simulink model "SG__MDL_LOG_ISSUE"  (R2022b)
settings: Solver=FixedStepAuto  StartTime=0.0  StopTime=Inf  FixedStep=ts  RelTol=1e-3  EnableMultiTasking=on
model workspace (MAT data in the model file):
  N_trig = Simulink.Parameter
  N_trig.Value = 4
  N_trig.Description = 'number of samples for triggered pulse for recording'
  N_trig.DataType = 'auto'
  N_trig.Complexity = 'real'
  N_trig.Dimensions = [1 1]
  Sig = Simulink.Signal
  Sig.DataType = 'auto'
  Sig.Dimensions = -1
  Sig.DimensionsMode = 'auto'
  Sig.Complexity = 'auto'
  Sig.SampleTime = -1
  Sig.SamplingMode = 'auto'
  dtf_a = Simulink.Parameter
  dtf_a.Value = [1  1  1; 1  1  1; 1  1  1; 1  1  1; 1  1  1; 1  1  1; 1  1  1; 1  1  1; 1  1  1; 1  1  1; 1  1  1; 1  1  1; 1  1  1; 1  1  1; 1  1  1; 1  1  1]
  dtf_a.DataType = 'auto'
  dtf_a.Complexity = 'real'
  dtf_a.Dimensions = [16 3]
  dtf_b = Simulink.Parameter
  dtf_b.Value = [0.5  0.5  0.5; 0.5  0.5  0.5; 0.5  0.5  0.5; 0.5  0.5  0.5; 0.5  0.5  0.5; 0.5  0.5  0.5; 0.5  0.5  0.5; 0.5  0.5  0.5; 0.5  0.5  0.5; 0.5  0.5  0.5; 0.5  0.5  0.5; 0.5  0.5  0.5; 0.5  0.5  0.5; 0.5  0.5  0.5; 0.5  0.5  0.5; 0.5  0.5  0.5]
  dtf_b.DataType = 'auto'
  dtf_b.Complexity = 'real'
  dtf_b.Dimensions = [16 3]
  enable_source = Simulink.Parameter
  enable_source.Value = 0
  enable_source.DataType = 'boolean'
  enable_source.Complexity = 'real'
  enable_source.Dimensions = [1 1]
  freq_fin = Simulink.Parameter
  freq_fin.Value = 1200
  freq_fin.DataType = 'auto'
  freq_fin.Complexity = 'real'
  freq_fin.Dimensions = [1 1]
  freq_ini = Simulink.Parameter
  freq_ini.Value = 150
  freq_ini.DataType = 'auto'
  freq_ini.Complexity = 'real'
  freq_ini.Dimensions = [1 1]
  k_L = Simulink.Parameter
  k_L.Value = [0; 0; 0; 0; 0; 0; 0; 0; 0; 0; 0; 0; 0; 0; 0; 0]
  k_L.Description = 'Coupling on left of ER. [Linear, NL]'
  k_L.DataType = 'auto'
  k_L.Complexity = 'real'
  k_L.Dimensions = [16 1]
  k_L_NL = Simulink.Parameter
  k_L_NL.Value = [0; 0; 0; 0; 0; 0; 0; 0; 0; 0; 0; 0; 0; 0; 0; 0]
  k_L_NL.Description = 'Coupling on left of ER. [Linear, NL]'
  k_L_NL.DataType = 'auto'
  k_L_NL.Complexity = 'real'
  k_L_NL.Dimensions = [16 1]
  k_O_NL = Simulink.Parameter
  k_O_NL.Value = [0; 0; 0; 0; 0; 0; 0; 0; 0; 0; 0; 0; 0; 0; 0; 0]
  k_O_NL.Description = 'Onsite nonlinearity'
  k_O_NL.DataType = 'auto'
  k_O_NL.Complexity = 'real'
  k_O_NL.Dimensions = [16 1]
  k_R = Simulink.Parameter
  k_R.Value = [0; 0; 0; 0; 0; 0; 0; 0; 0; 0; 0; 0; 0; 0; 0; 0]
  k_R.Description = 'Coupling on right of ER. [Linear, NL]'
  k_R.DataType = 'auto'
  k_R.Complexity = 'real'
  k_R.Dimensions = [16 1]
  k_R_NL = Simulink.Parameter
  k_R_NL.Value = [0; 0; 0; 0; 0; 0; 0; 0; 0; 0; 0; 0; 0; 0; 0; 0]
  k_R_NL.Description = 'Coupling on right of ER. [Linear, NL]'
  k_R_NL.DataType = 'auto'
  k_R_NL.Complexity = 'real'
  k_R_NL.Dimensions = [16 1]
  rec = Simulink.Parameter
  rec.Value = 1
  rec.DataType = 'boolean'
  rec.Complexity = 'real'
  rec.Dimensions = [1 1]
  src_select = Simulink.Parameter
  src_select.Value = 0
  src_select.DataType = 'auto'
  src_select.Complexity = 'real'
  src_select.Dimensions = [1 1]
  sweep_gain = Simulink.Parameter
  sweep_gain.Value = 0.02
  sweep_gain.DataType = 'auto'
  sweep_gain.Complexity = 'real'
  sweep_gain.Dimensions = [1 1]
  tmax = Simulink.Parameter
  tmax.Value = 10
  tmax.DataType = 'auto'
  tmax.Complexity = 'real'
  tmax.Dimensions = [1 1]
  ts_rec = Simulink.Parameter
  ts_rec.Value = 0.0001
  ts_rec.DataType = 'auto'
  ts_rec.Complexity = 'real'
  ts_rec.Dimensions = [1 1]
values from neighbouring files (symbols this model uses):
  ts = 400e-6    (= 0.0004)    [StartScript.m]
libraries: slrealtimeloglib x3, simulink x2, hdlsllib x2
settings Model: SimulationMode=external  ExplicitPartitioning=on  DataflowThreadingImplementation=Pthreads  Creator=padlewsk  LastModifiedBy=padlewsk
settings SolverCC: AllowMultiTaskInputOutput=on  ConcurrentTasks=on  AlgebraicLoopSolver=TrustRegion  PositivePriorityOrder=on  AutoInsertRateTranBlk=on
settings DataIOCC: SaveFormat=StructureWithTime
settings OptimizationCC: GainParamInheritBuiltInType=on  RollThreshold=33  EfficientFloat2IntCast=on  SimCompilerOptimization=on
settings DebuggingCC: TasksWithSamePriorityMsg=none  UnconnectedInputMsg=warning  UnconnectedOutputMsg=warning  UnconnectedLineMsg=warning  ModelReferenceSymbolNameMessage=none
settings HardwareCC: ProdBitPerLong=64  ProdLongLongMode=on  ProdHWDeviceType=Intel->x86-64 (Linux 64)
settings ModelReferenceCC: EnableRefExpFcnMdlSchedulingChecks=on
settings RTWCC: Description=Simulink Real-Time  SystemTargetFile=slrealtime.tlc  TemplateMakefile=slrealtime_default_tmf  Toolchain=Simulink Real-Time Toolchain  BuildConfiguration=Faster Runs  CodeExecutionProfiling=on  TargetLang=C++
settings SimulinkRealTimeTargetCC: UseGCCFastMath=on

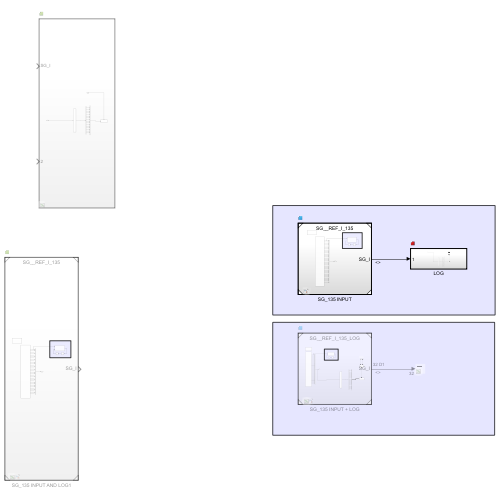
[thumbnail: Simulink's stored preview of the top-level diagram]
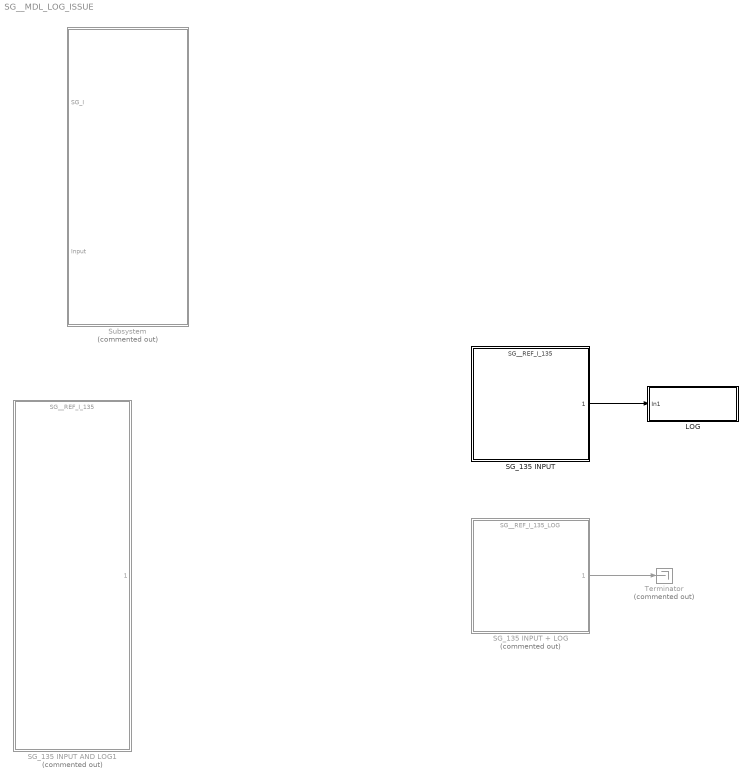
== system SG__MDL_LOG_ISSUE ==
  LOG : Subsystem  TreatAsAtomicUnit=on
  SG_135 INPUT : ModelReference  ModelNameDialog=SG__REF_I_135.slx  SimulationMode=Normal  ModelReferenceVersion=6.288
  SG_135 INPUT + LOG : ModelReference  Commented=on  ModelNameDialog=SG__REF_I_135_LOG.slx  SimulationMode=Normal  ModelReferenceVersion=6.291
  SG_135 INPUT AND LOG1 : ModelReference  Commented=on  ModelNameDialog=SG__REF_I_135.slx  SimulationMode=Normal  ModelReferenceVersion=6.288
  Subsystem : Subsystem  Commented=on  TreatAsAtomicUnit=on
  Terminator : Terminator  Commented=on
  wires:
  SG_135 INPUT/1 -> LOG/1(In1)
  SG_135 INPUT + LOG/1 -> Terminator/1

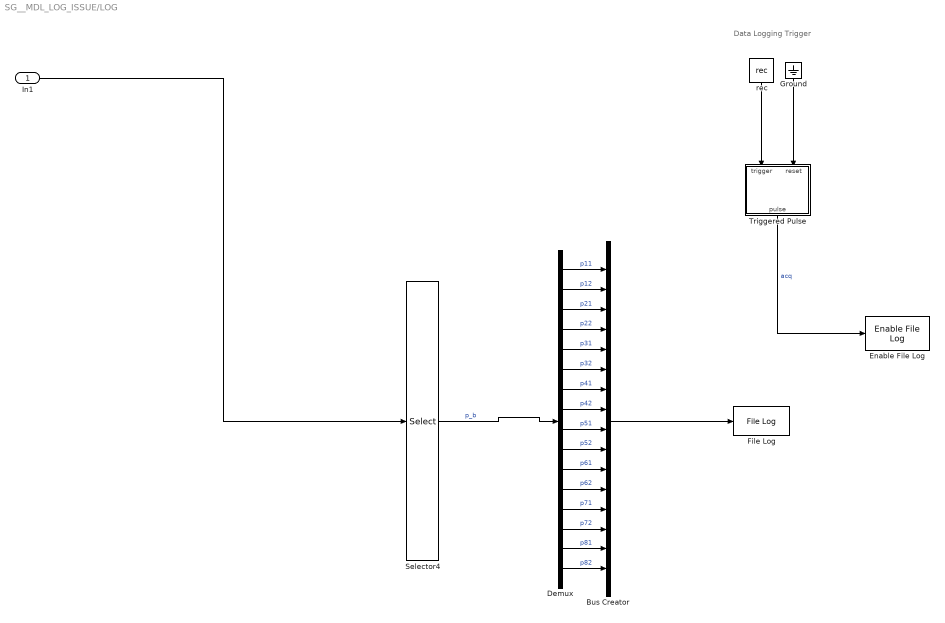
== system SG__MDL_LOG_ISSUE/LOG ==
  note: Data Logging Trigger
  In1 : Inport
  Bus Creator : BusCreator  Inputs=16
  Demux : Demux  Outputs=16
  Enable File Log : slrealtimeloglib/Enable File Log
  File Log : slrealtimeloglib/File Log  decimation=1  inputProcessing=Elements as channels (sample based)
  Ground : Ground
  Selector4 : Selector  InputPortWidth=32  IndexOptions=Index vector (dialog)  Indices=[1:2:32]  OutputSizes=1
  "Triggered Pulse " : Subsystem  TreatAsAtomicUnit=on  mask(Triggered Pulse){N=3000}
      mask prompts: N "Length (N samples)"
      mask help: Generates a single pulse of N samples length
  rec : Constant  Value=rec  SampleTime=-1
  wires:
  Demux/14 -> Bus Creator/14  "p72"
  Demux/10 -> Bus Creator/10  "p52"
  Demux/13 -> Bus Creator/13  "p71"
  Demux/11 -> Bus Creator/11  "p61"
  Demux/5 -> Bus Creator/5  "p31"
  Demux/4 -> Bus Creator/4  "p22"
  Selector4/1 -> Demux/1  "p_b"
  Demux/3 -> Bus Creator/3  "p21"
  Demux/16 -> Bus Creator/16  "p82"
  Demux/6 -> Bus Creator/6  "p32"
  Demux/9 -> Bus Creator/9  "p51"
  Demux/12 -> Bus Creator/12  "p62"
  Demux/2 -> Bus Creator/2  "p12"
  rec/1 -> "Triggered Pulse "/1(trigger)
  Bus Creator/1 -> File Log/1
  In1/1 -> Selector4/1
  Demux/8 -> Bus Creator/8  "p42"
  Ground/1 -> "Triggered Pulse "/2(reset)
  Demux/15 -> Bus Creator/15  "p81"
  Demux/7 -> Bus Creator/7  "p41"
  Demux/1 -> Bus Creator/1  "p11"
  "Triggered Pulse "/1(pulse) -> Enable File Log/1  "acq"

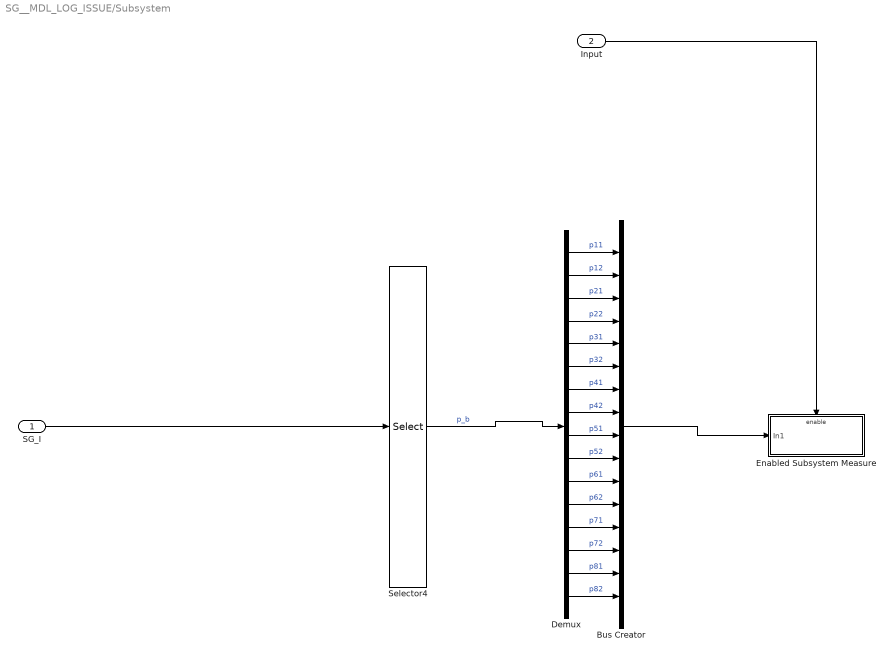
== system SG__MDL_LOG_ISSUE/Subsystem ==
  SG_I : Inport  SampleTime=ts
  Input : Inport  Port=2  OutDataTypeStr=boolean
  Bus Creator : BusCreator  Inputs=16
  Demux : Demux  Outputs=16
  Enabled Subsystem Measure : Subsystem
  Selector4 : Selector  InputPortWidth=32  IndexOptions=Index vector (dialog)  Indices=[1:2:32]  OutputSizes=1
  wires:
  Demux/15 -> Bus Creator/15  "p81"
  Bus Creator/1 -> Enabled Subsystem Measure/1(In1)
  Demux/9 -> Bus Creator/9  "p51"
  Demux/12 -> Bus Creator/12  "p62"
  Demux/1 -> Bus Creator/1  "p11"
  Demux/16 -> Bus Creator/16  "p82"
  Demux/8 -> Bus Creator/8  "p42"
  Demux/11 -> Bus Creator/11  "p61"
  Demux/2 -> Bus Creator/2  "p12"
  Demux/7 -> Bus Creator/7  "p41"
  Demux/10 -> Bus Creator/10  "p52"
  Demux/5 -> Bus Creator/5  "p31"
  Demux/13 -> Bus Creator/13  "p71"
  Demux/14 -> Bus Creator/14  "p72"
  Demux/4 -> Bus Creator/4  "p22"
  Demux/6 -> Bus Creator/6  "p32"
  Demux/3 -> Bus Creator/3  "p21"
  Selector4/1 -> Demux/1  "p_b"
  SG_I/1 -> Selector4/1
  Input/1 -> Enabled Subsystem Measure/Enable

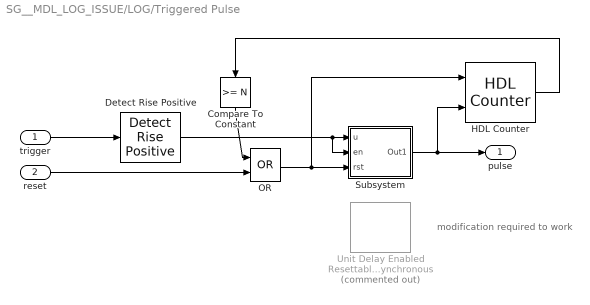
== system SG__MDL_LOG_ISSUE/LOG/Triggered Pulse  ==
  note: modification required to work
  trigger : Inport
  reset : Inport  Port=2
  Compare To Constant : simulink/Logic and Bit Operations/Compare To Constant  relop=>=  const=N  OutDataTypeStr=boolean
  Detect Rise Positive : simulink/Logic and Bit Operations/Detect Rise Positive  vinit=0  OutDataTypeStr=boolean
  HDL Counter : hdlsllib/Sources/HDL Counter  CountType=Free running  CountInit=1  CountStep=1  CountMax=25  CountFromType=Initial value  CountFrom=1  CountResetPort=on  CountLoadPort=off  CountEnbPort=on  CountDirPort=off  CountHitOutputPort=off  CountDataType=Unsigned  CountWordLen=32  CountFracLen=0  CountSampTime=1
  OR : Logic  Operator=OR  AllPortsSameDT=off  OutDataTypeStr=boolean
  Subsystem : Subsystem
  Unit Delay Enabled Resettable Synchronous : hdlsllib/Discrete/Unit Delay Enabled Resettable Synchronous  Commented=on  InitialCondition=0.0  SampleTime=-1
  pulse : Outport  VectorParamsAs1DForOutWhenUnconnected=off
  wires:
  OR/1 -> Subsystem/3(rst), HDL Counter/1
  trigger/1 -> Detect Rise Positive/1
  Subsystem/1(Out1) -> HDL Counter/2, pulse/1
  Compare To Constant/1 -> OR/1
  reset/1 -> OR/2
  Detect Rise Positive/1 -> Subsystem/2(en), Subsystem/1(u)
  HDL Counter/1 -> Compare To Constant/1

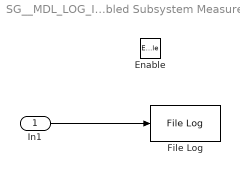
== system SG__MDL_LOG_ISSUE/Subsystem/Enabled Subsystem Measure ==
  In1 : Inport
  Enable : EnablePort
  File Log : slrealtimeloglib/File Log  decimation=1  inputProcessing=Elements as channels (sample based)
  wires:
  In1/1 -> File Log/1

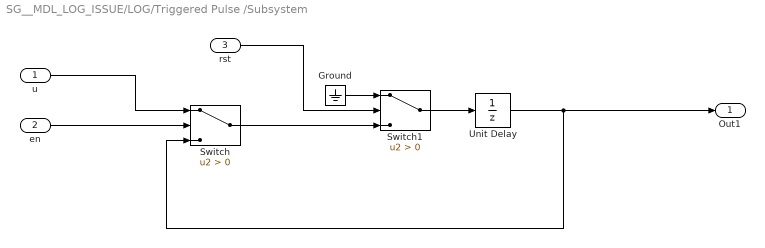
== system SG__MDL_LOG_ISSUE/LOG/Triggered Pulse /Subsystem ==
  u : Inport
  en : Inport  Port=2
  rst : Inport  Port=3
  Ground : Ground
  Switch : Switch  Criteria=u2 > Threshold  SaturateOnIntegerOverflow=off  InputSameDT=off
  Switch1 : Switch  Criteria=u2 > Threshold  SaturateOnIntegerOverflow=off  InputSameDT=off
  Unit Delay : UnitDelay  SampleTime=-1  HasFrameUpgradeWarning=on
  Out1 : Outport
  wires:
  Unit Delay/1 -> Switch/3, Out1/1
  en/1 -> Switch/2
  u/1 -> Switch/1
  rst/1 -> Switch1/2
  Ground/1 -> Switch1/1
  Switch1/1 -> Unit Delay/1
  Switch/1 -> Switch1/3
